simulink model "verify_Flow_Mixer_Thermostatic_mdl_new"  (R2018b)
settings: Solver=ode45  StartTime=0.0  StopTime=600  MaxStep=1  RelTol=1e-3  EnableMultiTasking=on
undefined symbols (not defined in the file or in its folder): path_carnot
libraries: carnot x7, simulink x2
settings Model: DEBUGGLOBALLEVEL=NOLEVEL  DEBUGMAXTOTALWARNINGS=inf  DEBUGMAXCONSECUTIVEWARNINGS=inf  DEBUGWRITETOFILE=0  DEBUGFILENAME='error.txt'  Creator=drhf  LastModifiedBy=P41573
settings DataIOCC: SaveFormat=Array  SignalLoggingSaveFormat=ModelDataLogs
settings OptimizationCC: ExpressionDepthLimit=2147483647  LifeSpan=inf
settings DebuggingCC: UnderspecifiedInitializationDetection=Classic  MergeDetectMultiDrivingBlocksExec=none  SolverPrmCheckMsg=warning  FcnCallInpInsideContextMsg=warning  StateNameClashWarn=warning  SFUnexpectedBacktrackingDiag=warning  SFNoUnconditionalDefaultTransitionDiag=warning  SFExecutionAtInitializationDiag=none
settings HardwareCC: ProdBitPerPointer=32  ProdBitPerSizeT=32  ProdBitPerPtrDiffT=32  ProdLargestAtomicFloat=None  ProdIntDivRoundTo=Undefined  ProdEndianess=Unspecified  ProdWordSize=32  ProdHWDeviceType=32-bit Generic
settings ModelReferenceCC: PropagateSignalLabelsOutOfModel=off
settings SFSimCC: SimUseLocalCustomCode=off
settings RTWCC: RTWUseLocalCustomCode=off
settings CodeAppCC: StateflowObjectComments=on
settings GRTTargetCC: TargetLangStandard=C89/C90 (ANSI)  GeneratePreprocessorConditionals=Disable all  CombineOutputUpdateFcns=off  GRTInterface=on
settings ConfigComp: CovMetricSettings=dw  CovHtmlReporting=on  CovSaveCumulativeToWorkspaceVar=on  CovSaveSingleToWorkspaceVar=on  CovExternalEMLEnable=off

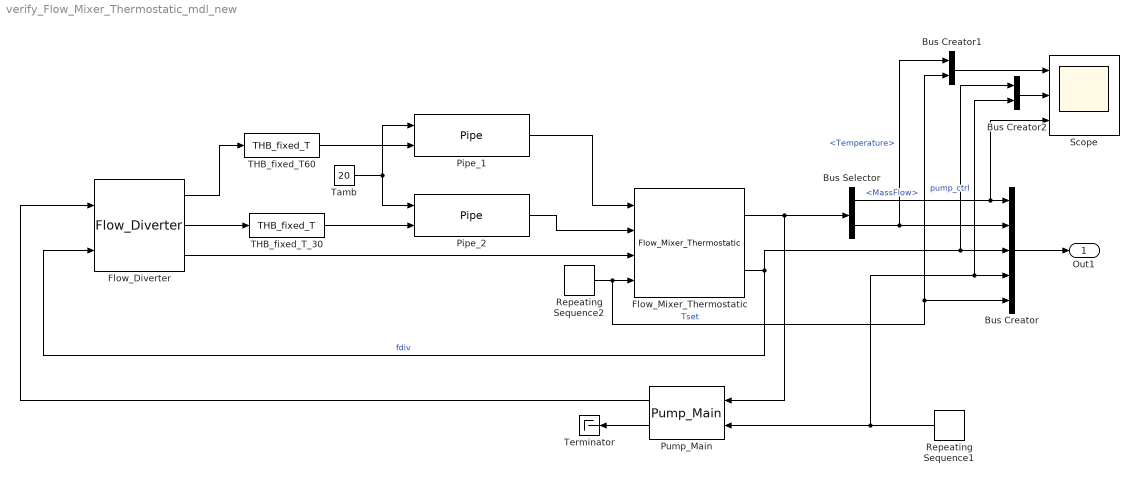
== system verify_Flow_Mixer_Thermostatic_mdl_new ==
  Bus Creator : BusCreator  Inputs=5
  Bus Creator1 : BusCreator  Inputs=2
  Bus Creator2 : BusCreator  Inputs=2
  Bus Selector : BusSelector  OutputSignals=MassFlow,Temperature
  Flow_Diverter : carnot/Hydraulics/Flow_Diverter
  Flow_Mixer_Thermostatic : carnot/Hydraulics/Flow_Mixer_Thermostatic  t=10
  Pipe_1 : carnot/Hydraulics/Pipe  dia=0.02  len=10  hgt=5  uloss=100/20/10  cond=0  cwall=1000  t0=20  lin=100/0.2  qua=100/0.2^2  nodes=10
  Pipe_2 : carnot/Hydraulics/Pipe  dia=0.02  len=10  hgt=5  uloss=100/20/10  cond=0  cwall=1000  t0=20  lin=100/0.2  qua=100/0.2^2  nodes=10
  Pump_Main : carnot/Hydraulics/Pump_Main  Tini=20  p0=3e5  IDpreset=pressure drop  fluid=Water  mix=0  mix2=0  mix3=0  t1=5  PathName=fullfile(path_carnot('libsl'), 'Hydraulics', 'Pump_Main', 'parameter_set')  FileName='Pump6m.mat'  userPath=off  userParam=off  a0=60000  a1=-43200  a2=0  dia=0.025  UA=1  mcp=4182  e0=50  e1=28.8  e2=-10.368
  Repeating Sequence1 : simulink/Sources/Repeating Sequence  rep_seq_t=[ 0 195 195.1 202 202.1 601]  rep_seq_y=[ 1 1 0 0 1 1]
  Repeating Sequence2 : simulink/Sources/Repeating Sequence  rep_seq_t=[0 300 350 601]  rep_seq_y=[50 50 35 35]
  Scope : Scope  NumInputPorts=3
  THB_fixed_T60 : carnot/Source/Simple/THB_fixed_T  t=60
  THB_fixed_T_30 : carnot/Source/Simple/THB_fixed_T  t=30
  Tamb : Constant  Value=20
  Terminator : Terminator
  Out1 : Outport
  wires:
  Bus Creator/1 -> Out1/1
  Flow_Mixer_Thermostatic/1 -> Pump_Main/1, Bus Selector/1
  Bus Selector/1 -> Scope/3, Bus Creator/1  "<MassFlow>"
  Bus Selector/2 -> Bus Creator1/1, Bus Creator/2  "<Temperature>"
  Flow_Mixer_Thermostatic/2 -> Flow_Diverter/2, Bus Creator2/1, Bus Creator/3  "fdiv"
  Tamb/1 -> Pipe_1/1, Pipe_2/1
  Pipe_1/1 -> Flow_Mixer_Thermostatic/1
  THB_fixed_T60/1 -> Pipe_1/2
  THB_fixed_T_30/1 -> Pipe_2/2
  Pipe_2/1 -> Flow_Mixer_Thermostatic/2
  Flow_Diverter/1 -> THB_fixed_T60/1
  Flow_Diverter/2 -> THB_fixed_T_30/1
  Flow_Diverter/3 -> Flow_Mixer_Thermostatic/3
  Repeating Sequence1/1 -> Pump_Main/2, Bus Creator2/2, Bus Creator/4  "pump_ctrl"
  Pump_Main/2 -> Terminator/1
  Pump_Main/1 -> Flow_Diverter/1
  Repeating Sequence2/1 -> Flow_Mixer_Thermostatic/4, Bus Creator/5, Bus Creator1/2  "Tset"
  Bus Creator1/1 -> Scope/1
  Bus Creator2/1 -> Scope/2
